simulink library "dynamicPressure_ul"  (R2020a)
settings: Solver=VariableStepAuto  StartTime=0.0  StopTime=10.0  RelTol=1e-3
settings Model: Creator=mcobb  LastModifiedBy=John Jr
settings DataIOCC: ReturnWorkspaceOutputs=off
settings DebuggingCC: ArithmeticOperatorsInVariantConditions=warning
settings SFSimCC: CustomCodeUndefinedFunction=UseInterfaceOnly

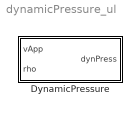
== system dynamicPressure_ul ==
  DynamicPressure : Subsystem  mask{rho=0}
      mask prompts: rho "Fluid density"

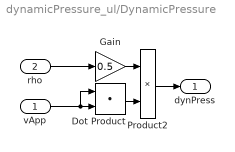
== system dynamicPressure_ul/DynamicPressure ==
  vApp : Inport
  rho : Inport  Port=2
  Dot Product : DotProduct  InputSameDT=on  OutDataTypeStr=Inherit: Inherit via internal rule
  Gain : Gain  Gain=0.5
  Product2 : Product
  dynPress : Outport  VectorParamsAs1DForOutWhenUnconnected=off
  wires:
  Product2/1 -> dynPress/1
  vApp/1 -> Dot Product/1, Dot Product/2
  rho/1 -> Gain/1
  Dot Product/1 -> Product2/2
  Gain/1 -> Product2/1
